simulink model "SSmodel"  (R2022b)
settings: Solver=VariableStepAuto  StartTime=0.0  StopTime=100  RelTol=1e-3
values from neighbouring files (symbols this model uses):
  A_value = A_optmse    [par_det_simulink.m]
  B_value = B_optmse    [par_det_simulink.m]
  C_value = C_optmse    [par_det_simulink.m]
  D_value = D_optmse    [par_det_simulink.m]
settings Model: Creator=niels  LastModifiedBy=remco

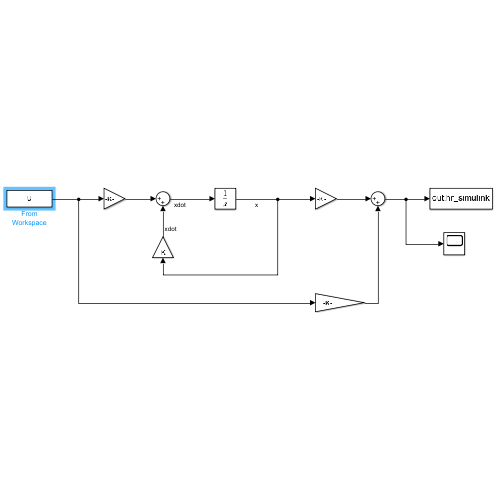
[thumbnail: Simulink's stored preview of the top-level diagram]
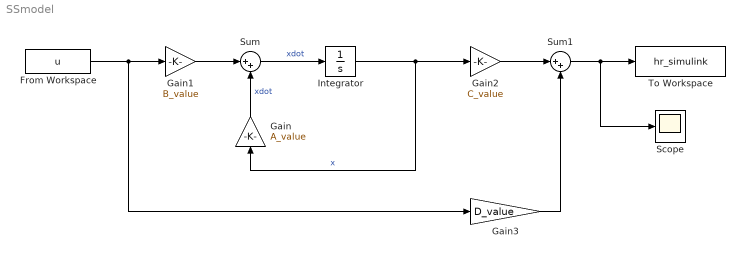
== system SSmodel ==
  From Workspace : FromWorkspace  VariableName=u  SampleTime=0.01
  Gain : Gain  Gain=A_value
  Gain1 : Gain  Gain=B_value
  Gain2 : Gain  Gain=C_value
  Gain3 : Gain  Gain=D_value
  Integrator : Integrator
  Scope : Scope
  Sum : Sum  Inputs=|++
  Sum1 : Sum  Inputs=|++
  To Workspace : ToWorkspace  VariableName=hr_simulink  SaveFormat=Structure With Time  SampleTime=-1
  wires:
  Sum/1 -> Integrator/1  "xdot"
  Integrator/1 -> Gain2/1, Gain/1  "x"
  Gain/1 -> Sum/2  "xdot"
  Gain1/1 -> Sum/1
  From Workspace/1 -> Gain3/1, Gain1/1
  Gain2/1 -> Sum1/1
  Gain3/1 -> Sum1/2
  Sum1/1 -> Scope/1, To Workspace/1
